simulink model "paletizadora"  (R2023b)
settings: Solver=ode4  StartTime=0.0  StopTime=100.0  FixedStep=0.04  RelTol=1e-3
libraries: simulink x6, slpidlib x2, Controllers x1
settings Model: Creator=root  LastModifiedBy=joallace

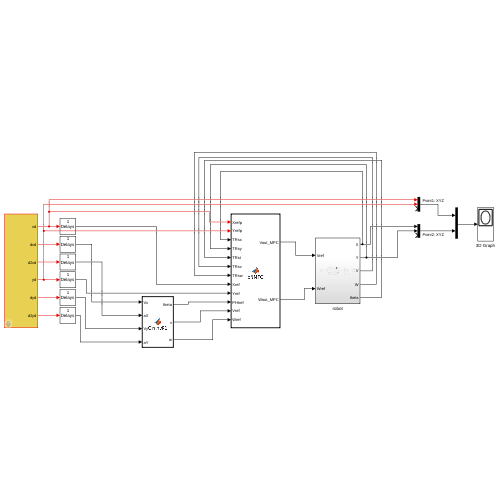
[thumbnail: Simulink's stored preview of the top-level diagram]
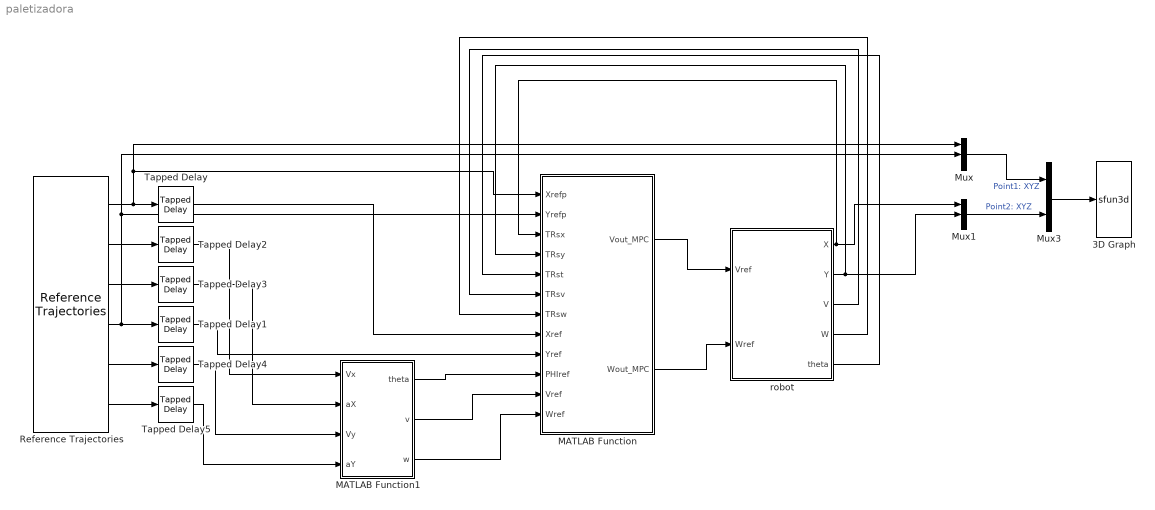
== system paletizadora ==
  3D Graph : S-Function  LoadFcn=if exist('sfun3d','file'), sfun3d([],[],[],'LoadBlock'); end  FunctionName=sfun3d  Parameters=ax,T,np,cp,gd,ls,mk,mx,hd,tb  SFunctionDeploymentMode=off  EnableBusSupport=off  mask(3D Graph){np=2, ax=[-4 4 -4 4 -3 3], mx=1e4, T=0.04, cp=[0 0 1], gd=on, hd=off, tb=on, ls=-, mk=none}
      mask prompts: np "Number of moving points (lines)"; ax "Range: [xmin xmax  ymin ymax zmin zmax]"; mx "Max number of points in each line"; T "Sampling Time"; cp "Camera position (use [0 0 1] for 2D XY view)"; gd "Grid (on|off)"; hd "HeadMarkers (on|off)"; tb "Toolbar (on|off)"; ls "LineStyle"; mk "LineMarker"
      mask help:
      | This block plots the position of several points in the XYZ space. The input contains the coordinates of all the points (x1,y1,z1,x2,y2,z2,...).
      | The number of moving points (lines), the XYZ ranges, sampling time, camera position, and grid (among other things) can be set as mask parameters.
      settings: CopyFcn=if exist('sfun3d','file'), sfun3d([],[],[],'CopyBlock'); end  DeleteFcn=if exist('sfun3d','file'), sfun3d([],[],[],'DeleteBlock'); end  NameChangeFcn=if exist('sfun3d','file'), sfun3d([],[],[],'NameChange'); end
      mask Help:
      | This block plots the position of several points in the XYZ space. The input contains the coordinates of all the points (x1,y1,z1,x2,y2,z2,...).
      | The number of moving points (lines), the XYZ ranges, sampling time, camera position, and grid (among other things) can be set as mask parameters.
      mask TypeOptions ls: - | -- | : | -. | none
      mask TypeOptions mk: none | . | + | o | * | x | square | diamond | v | ^ | > | < | pentagram | hexagram
      mask Display: plot([.05 .95 .95 .05 .05],[.45 .45 .95 .95 .45], 0.5+cos(0:0.1:2*pi)*0.3,0.7+sin(0:0.1:2*pi)*0.2)
  MATLAB Function : MATLAB Function  TreatAsAtomicUnit=on
  MATLAB Function1 : MATLAB Function  TreatAsAtomicUnit=on
  Mux : Mux  Inputs=3
  Mux1 : Mux  Inputs=3
  Mux3 : Mux  Inputs=2
  Reference Trajectories : Controllers/Reference Trajectories  trajectory_type=2  wf=0.10  raio_ref_1=1  delta_raio=0  t_delta_raio=60  xd=[1, -1.5]
  Tapped Delay{,1..5} (6 alike) : simulink/Discrete/Tapped Delay  vinit=0.0  samptime=-1  NumDelays=1  DelayOrder=Oldest  includeCurrent=off
  robot : Subsystem
  wires:
  MATLAB Function/1(Vout_MPC) -> robot/1(Vref)
  MATLAB Function/2(Wout_MPC) -> robot/2(Wref)
  Mux1/1 -> Mux3/2  "Point2: XYZ"
  Mux3/1 -> 3D Graph/1
  Mux/1 -> Mux3/1  "Point1: XYZ"
  robot/1(X) -> MATLAB Function/3(TRsx), Mux1/1
  robot/2(Y) -> MATLAB Function/4(TRsy), Mux1/2
  robot/3(V) -> MATLAB Function/6(TRsv)
  robot/4(W) -> MATLAB Function/7(TRsw)
  robot/5(theta) -> MATLAB Function/5(TRst)
  Reference Trajectories/1 -> MATLAB Function/1(Xrefp), Mux/1, Tapped Delay/1
  Tapped Delay/1 -> MATLAB Function/8(Xref)
  Reference Trajectories/4 -> Tapped Delay1/1, Mux/2, MATLAB Function/2(Yrefp)
  Tapped Delay1/1 -> MATLAB Function/9(Yref)
  Reference Trajectories/2 -> Tapped Delay2/1
  Reference Trajectories/3 -> Tapped Delay3/1
  Reference Trajectories/5 -> Tapped Delay4/1
  Reference Trajectories/6 -> Tapped Delay5/1
  Tapped Delay5/1 -> MATLAB Function1/4(aY)
  Tapped Delay4/1 -> MATLAB Function1/3(Vy)
  Tapped Delay3/1 -> MATLAB Function1/2(aX)
  Tapped Delay2/1 -> MATLAB Function1/1(Vx)
  MATLAB Function1/1(theta) -> MATLAB Function/10(PHIref)
  MATLAB Function1/3(w) -> MATLAB Function/12(Wref)
  MATLAB Function1/2(v) -> MATLAB Function/11(Vref)

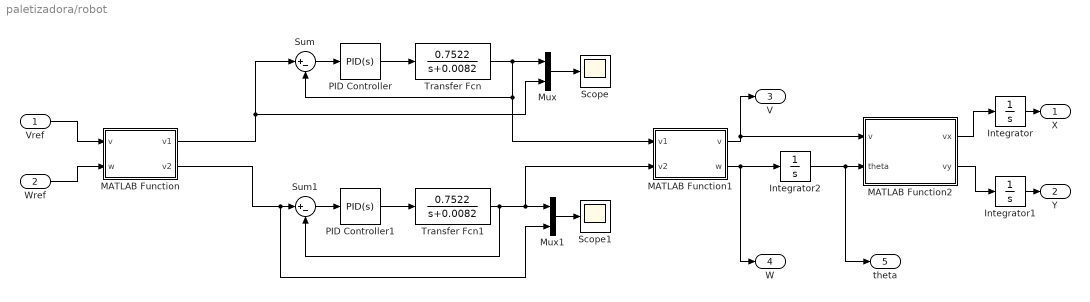
== system paletizadora/robot ==
  Vref : Inport
  Wref : Inport  Port=2
  Integrator : Integrator
  Integrator1 : Integrator
  Integrator2 : Integrator
  MATLAB Function : MATLAB Function  TreatAsAtomicUnit=on
  MATLAB Function1 : MATLAB Function  TreatAsAtomicUnit=on
  MATLAB Function2 : MATLAB Function  TreatAsAtomicUnit=on
  Mux : Mux  Inputs=2
  Mux1 : Mux  Inputs=2
  PID Controller : slpidlib/PID Controller  Controller=PID  Form=Ideal  TimeDomain=Continuous-time  UseExternalTs=off  SampleTime=-1  IntegratorMethod=Forward Euler  FilterMethod=Forward Euler  ControllerParametersSource=internal  P=34  I=3  UseKiTs=off  D=0  N=100  UseFilter=on  TunerSelectOption=Transfer Function Based (PID Tuner App)  InitialConditionSource=internal  InitialConditionForIntegrator=0  InitialConditionForFilter=0  DifferentiatorICPrevScaledInput=0  ExternalReset=none  TrackingMode=off  Kt=1  LimitOutput=off  SatLimitsSource=internal  UpperSaturationLimit=inf  LowerSaturationLimit=-inf  LinearizeAsGain=on  AntiWindupMode=none  Kb=1  LimitIntegrator=off  UpperIntegratorSaturationLimit=inf  LowerIntegratorSaturationLimit=-inf  POutMin=[]  POutMax=[]  IOutMin=[]  IOutMax=[]  DOutMin=[]  DOutMax=[]  NOutMin=[]  NOutMax=[]  SumOutMin=[]  SumOutMax=[]  SaturationOutMin=[]  SaturationOutMax=[]  PParamMin=[]  PParamMax=[]  IParamMin=[]  IParamMax=[]  DParamMin=[]  DParamMax=[]  NParamMin=[]  NParamMax=[]  KbParamMin=[]  KbParamMax=[]  KtParamMin=[]  KtParamMax=[]  KbOutMin=[]  KbOutMax=[]  KtOutMin=[]  KtOutMax=[]  IntegratorOutMin=[]  IntegratorOutMax=[]  FilterOutMin=[]  FilterOutMax=[]  SumI1OutMin=[]  SumI1OutMax=[]  SumI2OutMin=[]  SumI2OutMax=[]  SumI3OutMin=[]  SumI3OutMax=[]  SumI4OutMin=[]  SumI4OutMax=[]  SumDOutMin=[]  SumDOutMax=[]  DifferentiatorOutMin=[]  DifferentiatorOutMax=[]  FilterDiffOutCoefMin=[]  FilterDiffOutCoefMax=[]  ReciprocalOutMin=[]  ReciprocalOutMax=[]  SumDenOutMin=[]  SumDenOutMax=[]  SumNumOutMin=[]  SumNumOutMax=[]  DivideOutMin=[]  DivideOutMax=[]  UdiffTsProdOutMin=[]  UdiffTsProdOutMax=[]  NTsProdOutMin=[]  NTsProdOutMax=[]  UintegralTsProdOutMin=[]  UintegralTsProdOutMax=[]  UngainTsProdOutMin=[]  UngainTsProdOutMax=[]  ClampingZeroOutDataTypeStr=Inherit: Inherit via back propagation  ClampingZeroOutMin=[]  ClampingZeroOutMax=[]  FilterDenConstantOutDataTypeStr=Inherit: Inherit via back propagation  FilterDenConstantOutMin=[]  FilterDenConstantOutMax=[]  PCopyOutDataTypeStr=Inherit: Inherit via back propagation  PCopyOutMin=[]  PCopyOutMax=[]  NCopyOutDataTypeStr=Inherit: Inherit via back propagation  NCopyOutMin=[]  NCopyOutMax=[]  IntegratorContinuousStateAttributes=''  IntegratorStateMustResolveToSignalObject=off  IntegratorRTWStateStorageClass=Auto  FilterContinuousStateAttributes=''  FilterStateMustResolveToSignalObject=off  FilterRTWStateStorageClass=Auto  ParallelPVariant=Passthrough  IdealPVariant=InternalParameters  IVariant=InternalParameters  DVariant=InternalParameters  IntegratorVariant=Continuous  SatVariant=Disabled  AWVariant=Passthrough  PCopyVariant=Disabled  TRVariant=Disabled  FdbkBlocksVariant=Forward  IdealPFdbkVariant=Disabled  SatFdbkVariant=Disabled  DerivativeFilterVariant=ContFilter  NVariant=InternalParameters  NCopyVariant=Disabled  FilterICVariant=InternalICsFilter  IntegratorICVariant=InternalICs  ExternalResetVariant=Disabled  TRSumVariant=Passthrough  SumFdbkVariant=Disabled  SumVariant=Sum_PID  TsampFilterVariant=InternalTs  TsampNgainVariant=Passthrough  TsampIntegralVariant=Disabled_SignalSpec  ExternalSaturationOutDataTypeStr=Inherit: Same as second input
  PID Controller1 : slpidlib/PID Controller  Controller=PID  Form=Ideal  TimeDomain=Continuous-time  UseExternalTs=off  SampleTime=-1  IntegratorMethod=Forward Euler  FilterMethod=Forward Euler  ControllerParametersSource=internal  P=34  I=3  UseKiTs=off  D=0  N=100  UseFilter=on  TunerSelectOption=Transfer Function Based (PID Tuner App)  InitialConditionSource=internal  InitialConditionForIntegrator=0  InitialConditionForFilter=0  DifferentiatorICPrevScaledInput=0  ExternalReset=none  TrackingMode=off  Kt=1  LimitOutput=off  SatLimitsSource=internal  UpperSaturationLimit=inf  LowerSaturationLimit=-inf  LinearizeAsGain=on  AntiWindupMode=none  Kb=1  LimitIntegrator=off  UpperIntegratorSaturationLimit=inf  LowerIntegratorSaturationLimit=-inf  POutMin=[]  POutMax=[]  IOutMin=[]  IOutMax=[]  DOutMin=[]  DOutMax=[]  NOutMin=[]  NOutMax=[]  SumOutMin=[]  SumOutMax=[]  SaturationOutMin=[]  SaturationOutMax=[]  PParamMin=[]  PParamMax=[]  IParamMin=[]  IParamMax=[]  DParamMin=[]  DParamMax=[]  NParamMin=[]  NParamMax=[]  KbParamMin=[]  KbParamMax=[]  KtParamMin=[]  KtParamMax=[]  KbOutMin=[]  KbOutMax=[]  KtOutMin=[]  KtOutMax=[]  IntegratorOutMin=[]  IntegratorOutMax=[]  FilterOutMin=[]  FilterOutMax=[]  SumI1OutMin=[]  SumI1OutMax=[]  SumI2OutMin=[]  SumI2OutMax=[]  SumI3OutMin=[]  SumI3OutMax=[]  SumI4OutMin=[]  SumI4OutMax=[]  SumDOutMin=[]  SumDOutMax=[]  DifferentiatorOutMin=[]  DifferentiatorOutMax=[]  FilterDiffOutCoefMin=[]  FilterDiffOutCoefMax=[]  ReciprocalOutMin=[]  ReciprocalOutMax=[]  SumDenOutMin=[]  SumDenOutMax=[]  SumNumOutMin=[]  SumNumOutMax=[]  DivideOutMin=[]  DivideOutMax=[]  UdiffTsProdOutMin=[]  UdiffTsProdOutMax=[]  NTsProdOutMin=[]  NTsProdOutMax=[]  UintegralTsProdOutMin=[]  UintegralTsProdOutMax=[]  UngainTsProdOutMin=[]  UngainTsProdOutMax=[]  ClampingZeroOutDataTypeStr=Inherit: Inherit via back propagation  ClampingZeroOutMin=[]  ClampingZeroOutMax=[]  FilterDenConstantOutDataTypeStr=Inherit: Inherit via back propagation  FilterDenConstantOutMin=[]  FilterDenConstantOutMax=[]  PCopyOutDataTypeStr=Inherit: Inherit via back propagation  PCopyOutMin=[]  PCopyOutMax=[]  NCopyOutDataTypeStr=Inherit: Inherit via back propagation  NCopyOutMin=[]  NCopyOutMax=[]  IntegratorContinuousStateAttributes=''  IntegratorStateMustResolveToSignalObject=off  IntegratorRTWStateStorageClass=Auto  FilterContinuousStateAttributes=''  FilterStateMustResolveToSignalObject=off  FilterRTWStateStorageClass=Auto  ParallelPVariant=Passthrough  IdealPVariant=InternalParameters  IVariant=InternalParameters  DVariant=InternalParameters  IntegratorVariant=Continuous  SatVariant=Disabled  AWVariant=Passthrough  PCopyVariant=Disabled  TRVariant=Disabled  FdbkBlocksVariant=Forward  IdealPFdbkVariant=Disabled  SatFdbkVariant=Disabled  DerivativeFilterVariant=ContFilter  NVariant=InternalParameters  NCopyVariant=Disabled  FilterICVariant=InternalICsFilter  IntegratorICVariant=InternalICs  ExternalResetVariant=Disabled  TRSumVariant=Passthrough  SumFdbkVariant=Disabled  SumVariant=Sum_PID  TsampFilterVariant=InternalTs  TsampNgainVariant=Passthrough  TsampIntegralVariant=Disabled_SignalSpec  ExternalSaturationOutDataTypeStr=Inherit: Same as second input
  Scope : Scope
  Scope1 : Scope
  Sum : Sum  Inputs=|+-
  Sum1 : Sum  Inputs=|+-
  Transfer Fcn : TransferFcn  Numerator=[0.7522]  Denominator=[1 0.0082]
  Transfer Fcn1 : TransferFcn  Numerator=[0.7522]  Denominator=[1 0.0082]
  X : Outport
  Y : Outport  Port=2
  V : Outport  Port=3
  W : Outport  Port=4
  theta : Outport  Port=5
  wires:
  Sum/1 -> PID Controller/1
  PID Controller/1 -> Transfer Fcn/1
  Transfer Fcn/1 -> Sum/2, MATLAB Function1/1(v1), Mux/1
  Mux/1 -> Scope/1
  MATLAB Function/1(v1) -> Sum/1, Mux/2
  Transfer Fcn1/1 -> Sum1/2, MATLAB Function1/2(v2), Mux1/1
  Mux1/1 -> Scope1/1
  PID Controller1/1 -> Transfer Fcn1/1
  Sum1/1 -> PID Controller1/1
  Vref/1 -> MATLAB Function/1(v)
  Wref/1 -> MATLAB Function/2(w)
  MATLAB Function/2(v2) -> Mux1/2, Sum1/1
  MATLAB Function1/1(v) -> V/1, MATLAB Function2/1(v)
  MATLAB Function1/2(w) -> Integrator2/1, W/1
  Integrator2/1 -> MATLAB Function2/2(theta), theta/1
  MATLAB Function2/1(vx) -> Integrator/1
  MATLAB Function2/2(vy) -> Integrator1/1
  Integrator1/1 -> Y/1
  Integrator/1 -> X/1

== matlab function paletizadora/robot/MATLAB Function1 ==
  data: v1 input; v output; v2 input; w output
function [v,w] = CinDir(v1,v2)

l = 0.177;

v = (v1 + v2)/2;
w = (v1 - v2)/l;

== matlab function paletizadora/robot/MATLAB Function ==
  data: v input; v1 output; w input; v2 output
function [v1, v2] = CinInv(v,w)

l = 0.177;

v1 = (2*v + w*l)/2;
v2 = (2*v - w*l)/2;

== matlab function paletizadora/robot/MATLAB Function2 ==
  data: v input; vx output; theta input; vy output
function [vx, vy] = CinDirP2(v, theta)

vx = v*cos(theta);
vy = v*sin(theta);

== matlab function paletizadora/MATLAB Function ==
  data: Xrefp input; Vout_MPC output; Yrefp input; TRsx input; TRsy input; TRst input; TRsv input; TRsw input; Xref input; Yref input; PHIref input; Vref input; Wref input; Wout_MPC output
function [Vout_MPC,Wout_MPC]=cNMPC(Xrefp,Yrefp,TRsx,TRsy,...
    TRst,TRsv,TRsw,Xref,Yref,PHIref,Vref,Wref)
    
    Vmax=0.4;
    d=0.177;
    N1=1;
    N2=10;
    Nu=2;
    L1=10;
    L2=2000;
    L3=0.05;
    eta=0.1;
    Imax=15;
    I=0;
    Delta=0.1;
    
    alpha=0.015;
    
    Jsteps = zeros((Nu*4),1);
    Jgrad = zeros((Nu*2),1);
    Jgrad_prev = zeros((Nu*2),1);
    
    Ubest = zeros(2,Nu);
    Uref = zeros(2,Nu);
    Uaux = zeros(2,Nu);
    
    SimRob=struct('x',0,'y',0,'teta',0,'v',0,'w',0);
    
    for l=1:1:Nu
        Uref(1,l) = Vref;
        Uref(2,l) = Wref;
    end
    
    lTi = 0;
    [tPX,tPY,tPTeta]=calcRefTraj(lTi,TRsx,TRsy,TRst,Xref,Yref,PHIref,Vref,Wref,N2,Xrefp,Yrefp);
    tPXa=tPX(1);
    tPYa=tPY(1);
    tPTa=tPTeta(1);
    
    SimRob.x=TRsx;
    SimRob.y=TRsy;
    SimRob.teta=TRst;
    SimRob.v=TRsv;
    SimRob.w=TRsw;
    
    % SATURA AS VELOCIDADES DAS RODAS BASEADO NA VELOCIDADE MÁXIMA
    Uref=scaleForSaturation(Uref,d,Nu,Vmax);
    
    % CALCULA O VALOR INICIAL DA FUNÇÃO CUSTO J
    Jatual=COST_FUNCTION2(SimRob.x,SimRob.y,SimRob.teta,SimRob.v,SimRob.w,Uref,tPX,tPY,tPTeta,N1,N2,Nu,L1,L2,L3);
    Jbest = Jatual;
    
    while (I<Imax)&&(Jatual>eta)
        Usteps=calcUsteps(Uref,Nu,Delta);
        for k=0:1:Nu-1
            for j=1:1:4
                for m=0:1:Nu-1
                    if m==k
                        Uaux(1,m+1)=Usteps(1,(j+4*k));
                        Uaux(2,m+1)=Usteps(2,(j+4*k));
                    else
                        Uaux(1,m+1)=Uref(1,1);
                        Uaux(2,m+1)=Uref(2,1);
                    end
                end
    
                SimRob.x=TRsx;
                SimRob.y=TRsy;
                SimRob.teta=TRst;
                SimRob.v=TRsv;
                SimRob.w=TRsw;
    
                Uaux = scaleForSaturation(Uaux, d, Nu, Vmax);
    
                J=COST_FUNCTION2(SimRob.x,SimRob.y,SimRob.teta,SimRob.v,SimRob.w,Uaux,tPX,tPY,tPTeta,N1,N2,Nu,L1,L2,L3);
                Jsteps(j+4*k,1)=J;
    
            end
        end
    
        for h=0:1:Nu-1
            Jgrad_prev(2*h+1,1)=Jgrad(2*h+1,1);
            Jgrad(2*h+1,1)=Jsteps(4*h+1,1)-Jsteps(4*h+2,1);
            Jgrad_prev(2*h+2,1)=Jgrad(2*h+2,1);
            Jgrad(2*h+2,1)=Jsteps(4*h+3,1)-Jsteps(4*h+4,1);
        end
    
        di=[0 0];
        x1=di;
        for z=0:1:Nu-1
            di(1)=Jgrad(2*z+1,1);
            di(2)=Jgrad(2*z+2,1);
            x1(1)=(Uref(1,z+1) - alpha*di(1));
            x1(2)=(Uref(2,z+1) - alpha*di(2));
            Jgrad_prev(2*z+1,1)=Jgrad(2*z+1,1);
            Jgrad(2*z+1,1)=Jsteps(4*z+1,1)-Jsteps(4*z+2,1);
            Jgrad_prev(2*z+2,1)=Jgrad(2*z+2,1);
            Jgrad(2*z+2,1)=Jsteps(4*z+3,1)-Jsteps(4*z+4,1);
            beta=0;
            if ((Jgrad(2*z+1,1)>=eta)||(Jgrad(2*z+2,1)>=eta))
                t1=(Jgrad(2*z+1,1)-Jgrad_prev(2*z+1,1));
                t2=(Jgrad(2*z+2,1)-Jgrad_prev(2*z+2,1));
                a1=(Jgrad(2*z+1,1)*t1);
                a2=(Jgrad(2*z+2,1)*t2);
                b1=(Jgrad_prev(2*z+1,1)*Jgrad_prev(2*z+1,1));
                b2=(Jgrad_prev(2*z+2,1)*Jgrad_prev(2*z+2,1));
                beta=((a1+a2)/(b1+b2));
            end
            Uref(1,z+1)=x1(1)+alpha*(-Jgrad(2*z+1,1)+beta*Jgrad_prev(2*z+1,1));
            Uref(2,z+1)=x1(2)+alpha*(-Jgrad(2*z+2,1)+beta*Jgrad_prev(2*z+2,1));
        end
        SimRob.x=TRsx;
        SimRob.y=TRsy;
        SimRob.teta=TRst;
        SimRob.v=TRsv;
        SimRob.w=TRsw;
        
        % SATURA AS VELOCIDADES DAS RODAS BASEADO NA VELOCIDADE MÁXIMA
        Uref=scaleForSaturation(Uref,d,Nu,Vmax);
        Jatual=COST_FUNCTION2(SimRob.x,SimRob.y,SimRob.teta,SimRob.v,SimRob.w,Uref,tPX,tPY,tPTeta,N1,N2,Nu,L1,L2,L3);
        %TESTA SE O J ENCONTRADO É MELHOR QUE O J ANTERIOR
        if Jatual < Jbest
            Jbest = Jatual;
            Ubest = Uref;
        end
        I=I+1;

    end

    Vout_MPC = Ubest(1,1);
    Wout_MPC = Ubest(2,1);
end

== matlab function paletizadora/MATLAB Function1 ==
  data: theta output; Vx input; v output; aX input; Vy input; w output; aY input
function [theta, v, w] = CinInvP1(Vx, aX, Vy, aY)
theta = atan2(Vy,Vx);
v = sqrt(Vx^2+Vy^2);
w = (Vx*aY - Vy*aX)/(Vx^2+Vy^2);
